simulink model "SM"  (R2023b)
settings: Solver=VariableStepDiscrete  StartTime=0.0  StopTime=2  RelTol=1e-4
values from neighbouring files (symbols this model uses):
  C_PM = 1.758e-3    (= 0.001758)    [HVDCMMCInterconnectionParam.m]
  HRM = 2    [HVDCMMCInterconnectionParam.m]
  L_cable = 15e-3    (= 0.015)    [HVDCMMCInterconnectionParam.m]
  R_cable = 0.5    [HVDCMMCInterconnectionParam.m]
  Tfault = 9999    [HVDCMMCInterconnectionParam.m]
  Ts = Ts_Control    (= 4e-05)    [HVDCMMCInterconnectionParam.m]
  Ts_Power = 20e-6    (= 2e-05)    [HVDCMMCInterconnectionParam.m]
  Vc0_PM = 0    [HVDCMMCInterconnectionParam.m]
  w = 2*pi*Fnom    (= 314.159265359)    [HVDCMMCInterconnectionParam.m]
undefined symbols (not defined in the file or in its folder): DiscIntNeverNeededParam, gcbh, sps_AC, sps_rtmsupport, sps_SM
libraries: simulink x4, spsControlledVoltageSourceLib x3, spsCurrentMeasurementLib x3, spsGroundLib x2, spsDiodeLib x2, spsVoltageMeasurementLib x1, spsThreePhaseSineGeneratorLib x1, spsSeriesRLCBranchLib x1, sps_lib x1
settings Model: Creator=rober  LastModifiedBy=rober

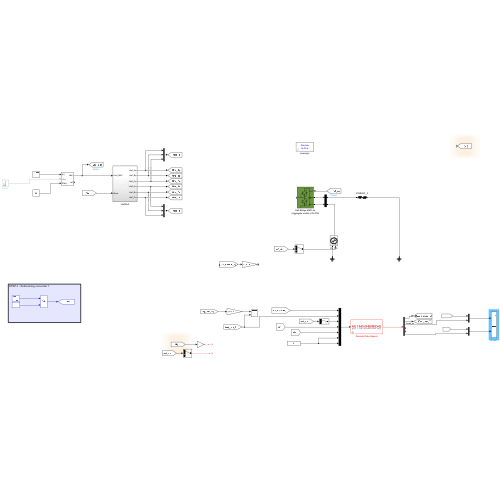
[thumbnail: Simulink's stored preview of the top-level diagram]
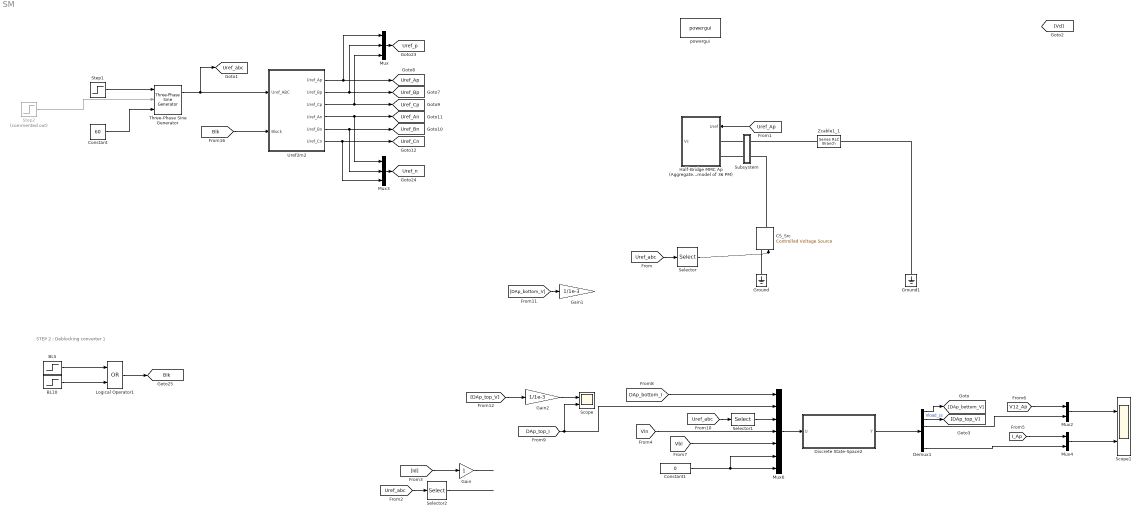
== system SM ==
  note: STEP 2 : Deblocking converter 1
  BL10 : Step  Time=Tfault+Ts_Power  SampleTime=Ts_Power
  BL5 : Step  Time=0.5  Before=1  After=0  SampleTime=Ts_Power
  CS_Src : spsControlledVoltageSourceLib/Controlled Voltage Source  Initialize=on  Source_Type=AC  Amplitude=0  Phase=0  Frequency=0  Measurements=None
  Constant : Constant  Value=60
  Constant1 : Constant  Value=0
  Demux1 : Demux  Outputs=numel(sps_SM.outputs)
  Discrete State-Space2 : Subsystem  SystemSampleTime=Ts_Power  mask{A=sps_SM.A, B=sps_SM.B, C=sps_SM.C, D=sps_SM.D, InitVec=sps_SM.x0, dt=Ts_Power, DQSYM=off, N=HRM, Ws=w}
      mask prompts: InitVec "Initial condition:"; dt "Time step (s):"; N "Harmonic number:"; Ws "Angular frequency (1/rad):"
      mask init:
      | % I = eye(size(A,1));
      | % INVR = I/(I-A*dt/2);
      | % Ad1 = INVR*(I+A*dt/2);
      | % Bd1 = INVR*B*dt/2;
      | % Cd1 = C*Ad1;
      | % Dd11 = C*INVR*B*dt/2+D;
      | % Dd12 = C*INVR*B*dt/2;
      | 
      |     I = eye(size(A,1));
      |     INVR = I/(I-A*dt/2);
      |     Ad1 = INVR*(I+A*dt/2);
      |     Bd1 = INVR*B;
      |     Cd1 = C*INVR*dt;
      |     Dd1 = Cd1*B/2 + D;
      | 
      | DQSYM = get_param(gcb,'DQSYM');
      | 
      | comp = 0;
      | 
      | if(strcmp(DQSYM,'on'))
      | 
      | %Calculating the PNZ matrices
      | 
      |     a = -0.5+0.866i;
      |     a2 = -0.5-0.866i;
      |     Sas = [1,a,a2;1,a2,a;1,1,1]/3;
      | 
      |     arows = size(Ad1,1)/3; %signal size
      |     acols = size(Ad1,2)/3; %signal size
      | 
      |     brows = size(Bd1,1)/3; %signal size
      |     bcols = size(Bd1,2)/3; %signal size
      | 
      |     crows = size(Cd1,1)/3; %signal size
      |     ccols = size(Cd1,2)/3; %signal size
      | 
      |     d1rows = size(Dd1,1)/3; %signal size
      |     d1cols = size(Dd1,2)/3; %signal size
      | 
      |     %%%%%%%%%%%%%%%%%%%%%%% Check for inconsistencies  %%%%%%%%%%%%%%%%%%%%%%%
      | 
      |     szMatA = size(A,1);
      |     iL = eye(szMatA);
      |     szMatiL = size(iL,1);
      | 
      |     if(szMatiL ~= szMatA || size(A,1) ~= size(A,2) || size(iL,1) ~= size(iL,2))
      |         error('[Int_DQN_Mat/swFeedback] check matrix A size!');
      |     end
      | 
      |     if(arows ~= brows || acols ~= ccols || crows ~= d1rows || bcols ~= d1cols)
      |         error('[Int_DQN_Mat/Initialize] the sizes of the state-space matrices!');
      |     end
      | 
      |     %%%%%%%%%%%%%%%%%%%%%%%%%%%%%%%%%%%%%%%%%%%%%%%%%%%%%%%%%%%%%%%
      | 
      | 
      |     %%%%%%%%%%%%%%%%%%%%%%% A --> Bpnz %%%%%%%%%%%%%%%%%%%%%%%
      |     Adc = complex(zeros(3*arows,3*acols));
      | 
      |     for i = 1 : arows
      |         for j = 1 : acols
      |             Adc((1:3) + (i-1)*3,(1:3) + (j-1)*3) = Sas*Ad1((1:3) + (i-1)*3,(1:3) + (j-1)*3)/Sas;
      |             %Adc((1:3) + (i-1)*3,(1:3) + (j-1)*3) = diag(diag(real(Adc((1:3) + (i-1)*3,(1:3) + (j-1)*3))));
      |             %Adc((1:3) + (i-1)*3,(1:3) + (j-1)*3) = diag(diag((Adc((1:3) + (i-1)*3,(1:3) + (j-1)*3))));
      | 
      |         end
      |     end
      |     %%%%%%%%%%%%%%%%%%%%%%%%%%%%%%%%%%%%%%%%%%%%%%%%%%%%%%%%%%%%%%%
      | 
      |     %%%%%%%%%%%%%%%%%%%%%%% B --> Bpnz %%%%%%%%%%%%%%%%%%%%%%%
      | 
      |     Bdc = complex(zeros(3*brows,3*bcols));
      | 
      |     for i = 1 : brows
      |         for j = 1 : bcols
      |             Bdc((1:3) + (i-1)*3,(1:3) + (j-1)*3) = Sas*Bd1((1:3) + (i-1)*3,(1:3) + (j-1)*3)/Sas;
      |             %Bdc((1:3) + (i-1)*3,(1:3) + (j-1)*3) = diag(diag(real(Bdc((1:3) + (i-1)*3,(1:3) + (j-1)*3))));
      |             %Bdc((1:3) + (i-1)*3,(1:3) + (j-1)*3) = diag(diag((Bdc((1:3) + (i-1)*3,(1:3) + (j-1)*3))));
      | 
      |         end
      |     end
      |     %%%%%%%%%%%%%%%%%%%%%%%%%%%%%%%%%%%%%%%%%%%%%%%%%%%%%%%%%%%%%%%
      | 
      |     %%%%%%%%%%%%%%%%%%%%%%% C --> Cpnz %%%%%%%%%%%%%%%%%%%%%%%
      | 
      |     Cdc = complex(zeros(3*crows,3*ccols));
      | 
      |     for i = 1 : crows
      |         for j = 1 : ccols
      |             Cdc((1:3) + (i-1)*3,(1:3) + (j-1)*3) = Sas*Cd1((1:3) + (i-1)*3,(1:3) + (j-1)*3)/Sas;
      |             %Cdc((1:3) + (i-1)*3,(1:3) + (j-1)*3) = diag(diag(real(Cdc((1:3) + (i-1)*3,(1:3) + (j-1)*3))));
      |             %Cdc((1:3) + (i-1)*3,(1:3) + (j-1)*3) = diag(diag((Cdc((1:3) + (i-1)*3,(1:3) + (j-1)*3))));
      |         end
      |     end
      |     %%%%%%%%%%%%%%%%%%%%%%%%%%%%%%%%%%%%%%%%%%%%%%%%%%%%%%%%%%%%%%%
      | 
      |     
      |     %%%%%%%%%%%%%%%%%%%%%%% D1 --> Cpnz %%%%%%%%%%%%%%%%%%%%%%%
      | 
      |     Ddc = complex(zeros(3*d1rows,3*d1cols));
      | 
      |     for i = 1 : d1rows
      |         for j = 1 : d1cols
      |             Ddc((1:3) + (i-1)*3,(1:3) + (j-1)*3) = Sas*Dd1((1:3) + (i-1)*3,(1:3) + (j-1)*3)/Sas;
      |             %Ddc1((1:3) + (i-1)*3,(1:3) + (j-1)*3) = diag(diag(real(Ddc1((1:3) + (i-1)*3,(1:3) + (j-1)*3))));
      |             %Ddc((1:3) + (i-1)*3,(1:3) + (j-1)*3) = diag(diag((Ddc((1:3) + (i-1)*3,(1:3) + (j-1)*3))));
      |         end
      |     end
      |     %%%%%%%%%%%%%%%%%%%%%%%%%%%%%%%%%%%%%%%%%%%%%%%%%%%%%%%%%%%%%%%
      | 
      |     Adc(abs(Adc)<2*eps) = 0;
      |     Bdc(abs(Bdc)<2*eps) = 0;
      |     Cdc(abs(Cdc)<2*eps) = 0;
      |     Ddc(abs(Ddc)<2*eps) = 0;
      | 
      |     InitVec_c = complex(zeros(brows*3,N+1));
      | 
      | 
      |     if(~isempty(InitVec))
      |         if(mod(numel(InitVec),3)~=0) 
      |             warning('[SS_DQNc_Mat] InitVec with wrong size --> needs to be a multiple of 3!'); 
      | 
      |         else
      |             for k = 1 : numel(InitVec)/3
      |                 InitVec_c((k-1)*3+1:(k-1)*3+3,1) = Sas*InitVec((k-1)*3+1:(k-1)*3+3)*exp(+1i*Ws*dt);
      |             end
      |         end
      |     end
      | 
      |     InitVec = InitVec_c;
      | 
      | 
      |     Ad1 = Adc;
      |     Bd1 = Bdc;
      |     Cd1 = Cdc;
      |     Dd1 = Ddc;
      | 
      |     comp = -1i*Ws*dt;
      | 
      | end
      settings: MinAlgLoopOccurrences=on
      settings: LibrarySourceBlock=|
      | spsSynchronousMachineModel/Discrete robust/State Space Model/Discretize
      | BE or Tustin
      mask Callback DQSYM:
      | EMT = get_param(gcb,'DQSYM');
      | 
      | if(strcmp(EMT,'on'))
      |    set_param(gcb,'MaskVisibilities',{'on','on','on','on','on','on','on','on','on'});
      | else
      |    set_param(gcb,'MaskVisibilities',{'on','on','on','on','on','on','on','off','off'});
      | end
      mask Display: disp(['{\color{red}\bf\fontsize{12}x(t) = Ad*x(t-dt)+Bd*u(t)}',newline,'{\color{gray}\bf\fontsize{12}y(t) = Cd*x(t-dt)+Dd*u(t)}'], 'texmode','on');
  Gain : Gain
  Gain1 : Gain  Gain=1/1e-3
  Gain2 : Gain  Gain=1/1e-3
  Ground : spsGroundLib/Ground  LConnTagsString=a
  Ground1 : spsGroundLib/Ground  LConnTagsString=a
  Half-Bridge MMC Ap (Aggregate model of 36 PM) : Subsystem  DialogController=POWERSYS.PowerSysDialog  LoadFcn=sps_rtmsupport('LoadFcn',gcbh);  StartFcn=sps_rtmsupport('StartFcn',gcbh);  StopFcn=sps_rtmsupport('StopFcn',gcbh);  mask(Half-Bridge MMC){ModelType=Aggregate model, n=36, C=C_PM, Vc_Initial=Vc0_PM, Ron=1e-3, Rs=1e6, Cs=inf, Ron_Diode=1e-1, Rs_Diode=1e3, Cs_Diode=inf, Vf_Diode=1e-3, Rs_CurrentSource=inf, Ts=Ts_Power}
      mask prompts: ModelType "Model type:"; n "Number of power modules"; C "Capacitor value (F)"; Vc_Initial "Capacitor initial voltage (V):"; Ron "Device on-state resistance (Ohms)"; Rs "Snubber resistance (Ohms)"; Cs "Snubber capacitance (F)"; Ron_Diode "Diode on-state resistance (Ohms)"; Rs_Diode "Diode snubber resistance (Ohms)"; Cs_Diode "Diode snubber capacitance (F)"; Vf_Diode "Diode forward voltage (V)"; Rs_CurrentSource "Current source snubber resistance (Ohms)"; Ts "Sample time (s):"
      mask help: Implements a half-bridge modular multilevel converter. The converter consists of multiple series-connected power modules. Each power module consists of one half-bridge and one capacitor on the DC side.
      mask init:
      | % block=gcb;
      | % [WantBlockChoice,Index1,MT,SPID] = powericon('FullBridgeMMCInit', block, ModelType, n, Ts, 2);
      | % powericon('SetInternalModels','set',block,WantBlockChoice);
      settings: LibrarySourceBlock=spsHalfBridgeMMCLib/Half-Bridge MMC  CopyFcn=sps_rtmsupport('CopyFcn',gcbh);  DeleteFcn=sps_rtmsupport('DeleteFcn',gcbh);  UndoDeleteFcn=sps_rtmsupport('UndoDeleteFcn',gcbh);  ModelCloseFcn=sps_rtmsupport('ModelCloseFcn',gcbh);  PreSaveFcn=sps_rtmsupport('PreSaveFcn',gcbh);  PostSaveFcn=sps_rtmsupport('PostSaveFcn',gcbh);  NameChangeFcn=sps_rtmsupport('NameChangeFcn',gcbh);  PreCopyFcn=sps_rtmsupport('PreCopyFcn',gcbh);  OpenFcn=sps_rtmsupport('OpenFcn',gcbh, [1]);  CloseFcn=sps_rtmsupport('CloseFcn',gcbh);  PreDeleteFcn=sps_rtmsupport('PreDeleteFcn',gcbh);
      mask Help: helpview(psbhelp);
      mask TypeOptions ModelType: Switching devices | Switching function | Average model (Uref-controlled) | Aggregate model
      mask Callback ModelType: powericon('FullBridgeMMCCback',gcb)
      mask Display:
      | x1=-0.04;
      | plot([0.5 0.80]+x1,[0.95 0.95])
      | plot([0.5 0.5]+x1,[0.95,0.80])
      | plot([0.5 0.38]+x1,[0.80 0.74])
      | plot([0.38 0.38]+x1,[0.80 0.62])
      | plot([0.38 0.5]+x1,[0.68 0.62])
      | plot([0.5 0.5]+x1,[0.62 0.52])
      | plot([0.45 0.5 0.43]+x1,[0.68 0.62 0.60])
      | %
      | y1=0.40;
      | plot([0.5 0.5]+x1,[0.95,0.80]-y1)
      | plot([0.5 0.38]+x1,[0.80 0.74]-y1)
      | plot([0.38 0.38]+x1,[0.80 0.62]-y1)
      | plot([0.38 0.5]+x1,[0.68 0.62]-y1)
      | plot([0.5 0.5]+x1,[0.62 0.52]-y1)
      | plot([0.45 0.5 0.43]+x1,[0.68 0.62 0.60]-y1)
      | plot([0.5 0.5]+x1,[0.2,0.10])
      | plot([0.5 0.80]+x1,[0.1 0.1])
      | %
      | plot([0.5 0.6]+x1,[0.84 0.84])
      | plot([0.6 0.6]+x1,[0.84 0.74])
      | plot([0.6 0.56]+x1,[0.74 0.69])
      | plot([0.6 0.64]+x1,[0.74 0.69])
      | plot([0.56 0.64]+x1,[0.69 0.69])
      | plot([0.6 0.6]+x1,[0.69 0.57])
      | plot([0.5 0.6]+x1,[0.57 0.57])
      | plot([0.55 0.65]+x1,[0.74 0.74])
      | %
      | y2=0.4;
      | plot([0.5 0.6]+x1,[0.84 0.84]-y2)
      | plot([0.6 0.6]+x1,[0.84 0.74]-y2)
      | plot([0.6 0.56]+x1,[0.74 0.69]-y2)
      | plot([0.6 0.64]+x1,[0.74 0.69]-y2)
      | plot([0.56 0.64]+x1,[0.69 0.69]-y2)
      | plot([0.6 0.6]+x1,[0.69 0.57]-y2)
      | plot([0.5 0.6]+x1,[0.57 0.57]-y2)
      | plot([0.55 0.65]+x1,[0.74 0.74]-y2)
      | %
      | plot([0.5 0.23]+x1,[0.5 0.5])
      | plot([0.23 0.23]+x1,[0.5 0.53])
      | plot([0.23 0.23]+x1,[0.55 0.58])
      | plot([0.23 0.23]+x1,[0.61 0.64])
      | %
      | plot([0.5 0.23]+x1,[0.1 0.1])
      | plot([0.23 0.23]+x1,[0.1 0.06])
      | plot([0.23 0.23]+x1,[0.04 0.01])
      | %
      | plot([0.34 0.34]+x1,[0.65 0.75])
      | plot([0.28 0.34]+x1,[0.7 0.7])
      | %
      | plot([0.34 0.34]+x1,[0.65 0.75]-y2)
      | plot([0.28 0.34]+x1,[0.7 0.7]-y2)
      | %
      | % Capacitor
      | plot([0.8 0.8]+x1,[0.51 0.95])
      | plot([0.72 0.88]+x1,[0.51 0.51])
      | plot([0.72 0.88]+x1,[0.51 0.51]-0.04)
      | plot([0.8 0.8]+x1,[0.47 0.1])
      | 
      | color('blue')
      | % switch lower(ModelType)
      | %     case 'average model (uref-controlled)'
      | %         port_label('input',1,'Uref')
      | %     case 'aggregate model'
      | %         port_label('input',1,'Uref')
      | %     otherwise
      | %         port_label('input',1,'Uref')
      | % end
      | port_label('output',1,'m')
  Logical Operator1 : Logic  Operator=OR  AllPortsSameDT=off  OutDataTypeStr=float('double')
  Mux : Mux  Inputs=3
  Mux2 : Mux  Inputs=2
  Mux3 : Mux  Inputs=3
  Mux4 : Mux  Inputs=2
  Mux6 : Mux  Inputs=numel(sps_SM.inputs)
  Scope : Scope  NumInputPorts=2
  Scope1 : Scope  NumInputPorts=2
  Selector : Selector  InputPortWidth=3  IndexOptions=Index vector (dialog)  Indices=1  OutputSizes=1
  Selector1 : Selector  InputPortWidth=3  IndexOptions=Index vector (dialog)  Indices=1  OutputSizes=1
  Selector2 : Selector  InputPortWidth=3  IndexOptions=Index vector (dialog)  Indices=1  OutputSizes=1
  Step1 : Step  Time=0.75  Before=60  After=100  SampleTime=Ts_Power
  Step2 : Step  Commented=on  Time=2.5  After=90  SampleTime=0
  Subsystem : Subsystem
  Three-Phase Sine Generator : spsThreePhaseSineGeneratorLib/Three-Phase Sine Generator  Ts=Ts_Power
      settings: LibrarySourceBlock=|
      | sps_lib/Sources/Signal Generator Sources/Three-Phase
      | Sine Generator
  Uref2m2 : Subsystem
  Zcable1_1 : spsSeriesRLCBranchLib/Series RLC Branch  LConnTagsString=__new0  RConnTagsString=__new0  BranchType=RL  Resistance=R_cable  Inductance=L_cable/3  SetiL0=off  InitialCurrent=0  Capacitance=1e-6  Setx0=off  InitialVoltage=0  Measurements=None
  powergui : sps_lib/powergui  Priority=1  SimulationMode=Discrete  SampleTime=Ts_Power  frequency=60  Iterations=50  frequencyindice=0  Pbase=100e6  ErrMax=1e-4  UnitsV=kV  UnitsW=MW  buscounter=0  FunctionMessages=off  echomessages=off  EnableUseOfTLC=off  CurrentSourceSwitches=off  DisableSnubberDevices=off  DisableRonSwitches=off  DisableVfSwitches=off  DisplayEquations=off  AutomaticDiscreteSolvers=off  SolverType=Tustin/Backward Euler (TBE)  Interpol=off  ExternalGateDelay=off  methode=off  Ts=100  x0status=blocks  SPID=on  SwTol=0  HookPort=off  NonlinearTolerance=1e-4  nMaxIteration=100  ContinueOnMaxIteration=off  RestoreLinks=warning  ResistiveCurrentMeasurement=off  Frange=[0:2:500]  Ylog=off  Xlog=on  ShowGrid=off  save=off  variable=ZData  structure=0  ZoomFFT=off  StartTime=0.0  cycles=1  DisplayStyle=1  fundamental=60  FreqAxis=off  MaxFrequency=1000  frequencyindicesteady=1  RmsSteady=1  display=off
  tag scope: Blk=global, Uref_An=global, Uref_Ap=global, Uref_Bn=global, Uref_Bp=global, Uref_Cn=global, Uref_Cp=global, Uref_abc=global, Uref_n=global, Uref_p=global
  wires:
  [Blk] -> Uref2m2/2(Block)
  Three-Phase Sine Generator/1 -> [Uref_abc], Uref2m2/1(Uref_ABC)
  Step1/1 -> Three-Phase Sine Generator/1
  Constant/1 -> Three-Phase Sine Generator/3
  Logical Operator1/1 -> [Blk]
  BL10/1 -> Logical Operator1/2
  BL5/1 -> Logical Operator1/1
  Uref2m2/6(Uref_Cn) -> Mux3/3, [Uref_Cn]
  Mux3/1 -> [Uref_n]
  Uref2m2/2(Uref_Bp) -> Mux/2, [Uref_Bp]
  Uref2m2/1(Uref_Ap) -> Mux/1, [Uref_Ap]
  Mux/1 -> [Uref_p]
  Uref2m2/5(Uref_Bn) -> Mux3/2, [Uref_Bn]
  Uref2m2/3(Uref_Cp) -> Mux/3, [Uref_Cp]
  Uref2m2/4(Uref_An) -> Mux3/1, [Uref_An]
  [Uref_abc] -> Selector/1
  Selector/1 -> CS_Src/1
  Step2/1 -> Three-Phase Sine Generator/2
  Mux2/1 -> Scope1/1
  Mux4/1 -> Scope1/2
  Mux6/1 -> Discrete State-Space2/1(U)
  Discrete State-Space2/1(Y) -> Demux1/1
  [Uref_Ap] -> Half-Bridge MMC Ap (Aggregate model of 36 PM)/1(Uref)
  Gain/1 -> ?
  [Id] -> Gain/1
  [Uref_abc] -> Selector2/1
  Selector2/1 -> ?
  Constant1/1 -> Mux6/6, Mux6/7
  [DAp_bottom_I] -> Mux6/1
  [DAp_top_I] -> Scope/2, Mux6/2
  [Uref_abc] -> Selector1/1
  [Vin] -> Mux6/4
  [Vbl] -> Mux6/5
  [I_Ap] -> Mux4/1
  Demux1/6 -> Mux4/2
  Demux1/3 -> Mux2/2
  [V12_Ap] -> Mux2/1
  Selector1/1 -> Mux6/3
  Demux1/2 -> [DAp_top_V]  "Vload_ss"
  Demux1/1 -> [DAp_bottom_V]
  [DAp_bottom_V] -> Gain1/1
  [DAp_top_V] -> Gain2/1
  Gain2/1 -> Scope/1
  connections:
  Ground/LConn1 -- CS_Src/LConn1
  Ground1/LConn1 -- Zcable1_1/LConn1
  Zcable1_1/RConn1 -- Subsystem/RConn1
  CS_Src/RConn1 -- Subsystem/RConn2
  Subsystem/LConn1 -- Half-Bridge MMC Ap (Aggregate model of 36 PM)/LConn1
  Subsystem/LConn2 -- Half-Bridge MMC Ap (Aggregate model of 36 PM)/LConn2

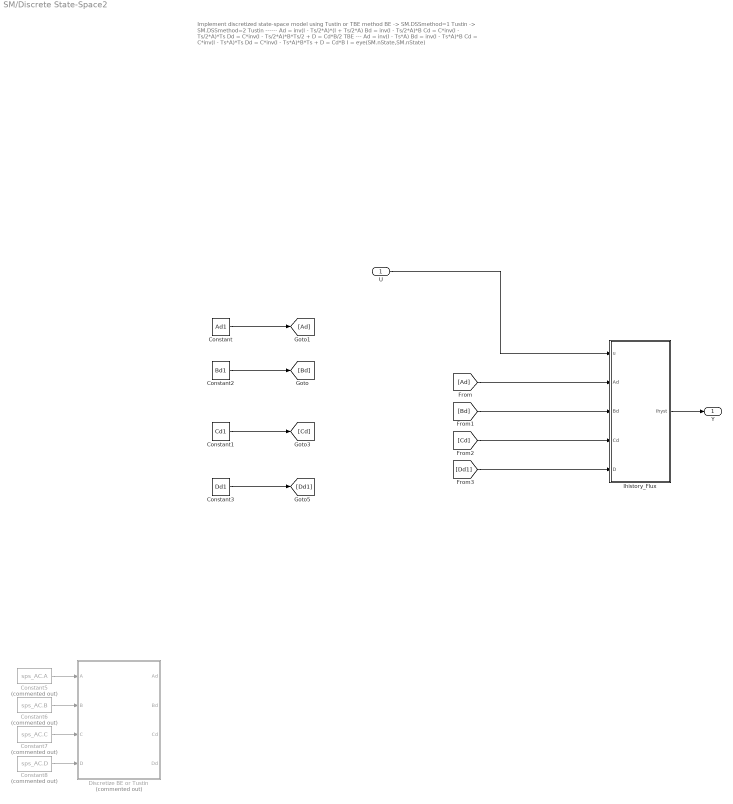
== system SM/Discrete State-Space2 ==
  note: Implement discretized state-space model using Tustin or TBE method
      |
      | BE      -> SM.DSSmethod=1
      | Tustin  -> SM.DSSmethod=2
      |
      |
      | Tustin
      | ------
      | Ad = inv(I - Ts/2*A)*(I + Ts/2*A)
      | Bd = inv(I - Ts/2*A)*B
      | Cd = C*inv(I - Ts/2*A)*Ts
      | Dd = C*inv(I - Ts/2*A)*B*Ts/2  + D  =  Cd*B/2
      |
      | TBE
      | ---
      | Ad = inv(I - Ts*A)
      | Bd = inv(I - Ts*A)*B
      | Cd = C*inv(I - Ts*A)*Ts
      | Dd = C*inv(I - Ts*A)*B*Ts  + D  =  Cd*B
      |
      | I = eye(SM.nState,SM.nState)
  U : Inport
  Constant : Constant  Value=Ad1
  Constant1 : Constant  Value=Cd1
  Constant2 : Constant  Value=Bd1
  Constant3 : Constant  Value=Dd1
  Constant5 : Constant  Commented=on  Value=sps_AC.A
  Constant6 : Constant  Commented=on  Value=sps_AC.B
  Constant7 : Constant  Commented=on  Value=sps_AC.C
  Constant8 : Constant  Commented=on  Value=sps_AC.D
  Discretize BE or Tustin : Subsystem  Commented=on  AncestorBlock="DQN_Machines/DQN_Mac_V1/Discretize  BE or Tustin"
  Ihistory_Flux : Subsystem  AncestorBlock=DQN_Machines/DQN_Mac_V1/Ihistory_Flux
  Y : Outport
  wires:
  Constant/1 -> [Ad]
  Constant2/1 -> [Bd]
  Constant1/1 -> [Cd]
  Constant3/1 -> [Dd1]
  Constant7/1 -> Discretize BE or Tustin/3(C)
  Constant6/1 -> Discretize BE or Tustin/2(B)
  Constant8/1 -> Discretize BE or Tustin/4(D)
  Constant5/1 -> Discretize BE or Tustin/1(A)
  U/1 -> Ihistory_Flux/1(u)
  Ihistory_Flux/1(Ihyst) -> Y/1
  [Ad] -> Ihistory_Flux/2(Ad)
  [Bd] -> Ihistory_Flux/3(Bd)
  [Cd] -> Ihistory_Flux/4(Cd)
  [Dd1] -> Ihistory_Flux/5(D)

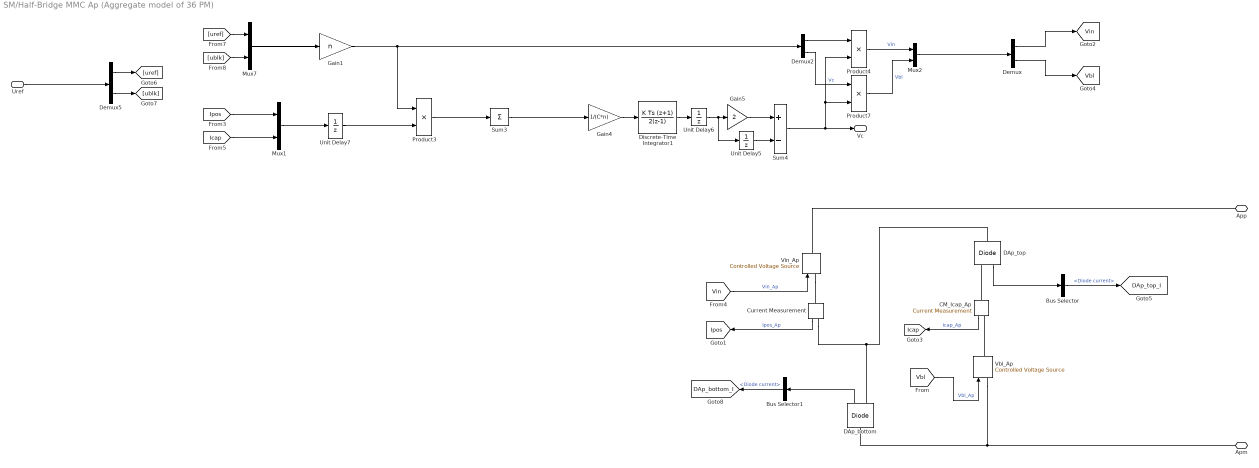
== system SM/Half-Bridge MMC Ap (Aggregate model of 36 PM) ==
  Uref : Inport
  Bus Selector : BusSelector  OutputSignals=Diode current
  Bus Selector1 : BusSelector  OutputSignals=Diode current
  CM_Icap_Ap : spsCurrentMeasurementLib/Current Measurement  PhasorSimulation=off  OutputType=Complex  PSBequivalent=0
  Current Measurement : spsCurrentMeasurementLib/Current Measurement  PhasorSimulation=off  OutputType=Complex  PSBequivalent=0
  DAp_bottom : spsDiodeLib/Diode  Ron=0.0001  Lon=0  Vf=0.0001  IC=0  UseSnubber=0  Rs=1e9  Cs=Cs_Diode  Measurements=on
  DAp_top : spsDiodeLib/Diode  Ron=0.0001  Lon=0  Vf=0.0001  IC=0  UseSnubber=0  Rs=1e9  Cs=Cs_Diode  Measurements=on
  Demux : Demux  Outputs=2
  Demux2 : Demux  Outputs=2
  Demux5 : Demux  Outputs=2
  Discrete-Time Integrator1 : DiscreteIntegrator  IntegratorMethod=Integration: Trapezoidal  gainval=1  InitialCondition=Vc_Initial  SampleTime=Ts  UpperSaturationLimit=5000  LowerSaturationLimit=500  ICPrevOutput=DiscIntNeverNeededParam  ICPrevScaledInput=DiscIntNeverNeededParam
  Gain1 : Gain  Gain=n
  Gain4 : Gain  Gain=1/(C*n)
  Gain5 : Gain  Gain=2
  Mux1 : Mux  Inputs=2
  Mux2 : Mux  Inputs=2
  Mux7 : Mux  Inputs=2
  Product3 : Product
  Product4 : Product
  Product7 : Product
  Sum3 : Sum  Inputs=1  InputSameDT=on  SaturateOnIntegerOverflow=on  OutDataTypeStr=Inherit: Same as first input
  Sum4 : Sum  Inputs=+-  InputSameDT=on  SaturateOnIntegerOverflow=on  OutDataTypeStr=Inherit: Same as first input
  Unit Delay5 : UnitDelay  InitialCondition=Vc_Initial  SampleTime=Ts  HasFrameUpgradeWarning=on
  Unit Delay6 : UnitDelay  InitialCondition=Vc_Initial  SampleTime=Ts  HasFrameUpgradeWarning=on
  Unit Delay7 : UnitDelay  SampleTime=Ts  HasFrameUpgradeWarning=on
  Vbl_Ap : spsControlledVoltageSourceLib/Controlled Voltage Source  Initialize=on  Source_Type=AC  Amplitude=0  Phase=0  Frequency=0  Measurements=None
  Vin_Ap : spsControlledVoltageSourceLib/Controlled Voltage Source  Initialize=on  Source_Type=AC  Amplitude=0  Phase=0  Frequency=0  Measurements=None
  App : PMIOPort  Side=Left
  Apm : PMIOPort  Port=2  Side=Left
  Vc : Outport  VectorParamsAs1DForOutWhenUnconnected=off
  tag scope: DAp_bottom_I=global, DAp_top_I=global, Icap=global, Ipos=global, Vbl=global, Vin=global
  wires:
  Demux/1 -> [Vin]
  [Vin] -> Vin_Ap/1  "Vin_Ap"
  Product3/1 -> Sum3/1
  Demux/2 -> [Vbl]
  [Ipos] -> Mux1/1
  Unit Delay5/1 -> Sum4/2
  Gain5/1 -> Sum4/1
  Sum4/1 -> Product7/2, Product4/2, Vc/1  "Vc"
  Discrete-Time Integrator1/1 -> Unit Delay6/1
  Mux2/1 -> Demux/1
  [Vbl] -> Vbl_Ap/1  "Vbl_Ap"
  [Icap] -> Mux1/2
  Gain4/1 -> Discrete-Time Integrator1/1
  Unit Delay6/1 -> Gain5/1, Unit Delay5/1
  Mux1/1 -> Unit Delay7/1
  Mux7/1 -> Gain1/1
  Demux2/1 -> Product4/1
  Demux2/2 -> Product7/1
  Product4/1 -> Mux2/1  "Vin"
  Product7/1 -> Mux2/2  "Vbl"
  Demux5/2 -> [ublk]
  [uref] -> Mux7/1
  [ublk] -> Mux7/2
  Current Measurement/1 -> [Ipos]  "Ipos_Ap"
  CM_Icap_Ap/1 -> [Icap]  "Icap_Ap"
  Unit Delay7/1 -> Product3/2
  Gain1/1 -> Demux2/1, Product3/1
  Demux5/1 -> [uref]
  Uref/1 -> Demux5/1
  Sum3/1 -> Gain4/1
  DAp_top/1 -> Bus Selector/1
  Bus Selector/1 -> [DAp_top_I]  "<Diode current>"
  DAp_bottom/1 -> Bus Selector1/1
  Bus Selector1/1 -> [DAp_bottom_I]  "<Diode current>"
  connections:
  Current Measurement/RConn1 -- DAp_bottom/RConn1 -- DAp_top/LConn1
  Apm/RConn1 -- Vbl_Ap/LConn1 -- DAp_bottom/LConn1
  Vbl_Ap/RConn1 -- CM_Icap_Ap/RConn1
  CM_Icap_Ap/LConn1 -- DAp_top/RConn1
  App/RConn1 -- Vin_Ap/RConn1
  Vin_Ap/LConn1 -- Current Measurement/LConn1

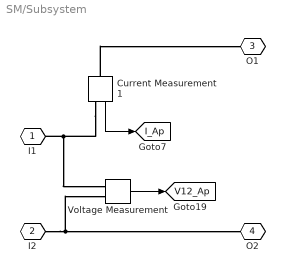
== system SM/Subsystem ==
  Current Measurement1 : spsCurrentMeasurementLib/Current Measurement  PhasorSimulation=off  OutputType=Complex  PSBequivalent=0
  Voltage Measurement : spsVoltageMeasurementLib/Voltage Measurement  PhasorSimulation=off  OutputType=Complex  PSBequivalent=0
  I1 : PMIOPort  Side=Left
  I2 : PMIOPort  Port=2  Side=Left
  O1 : PMIOPort  Port=3  Side=Right
  O2 : PMIOPort  Port=4  Side=Right
  tag scope: I_Ap=global, V12_Ap=global
  wires:
  Current Measurement1/1 -> [I_Ap]
  Voltage Measurement/1 -> [V12_Ap]
  connections:
  Current Measurement1/RConn1 -- Voltage Measurement/LConn1 -- I1/RConn1
  Current Measurement1/LConn1 -- O1/RConn1
  I2/RConn1 -- Voltage Measurement/LConn2 -- O2/RConn1

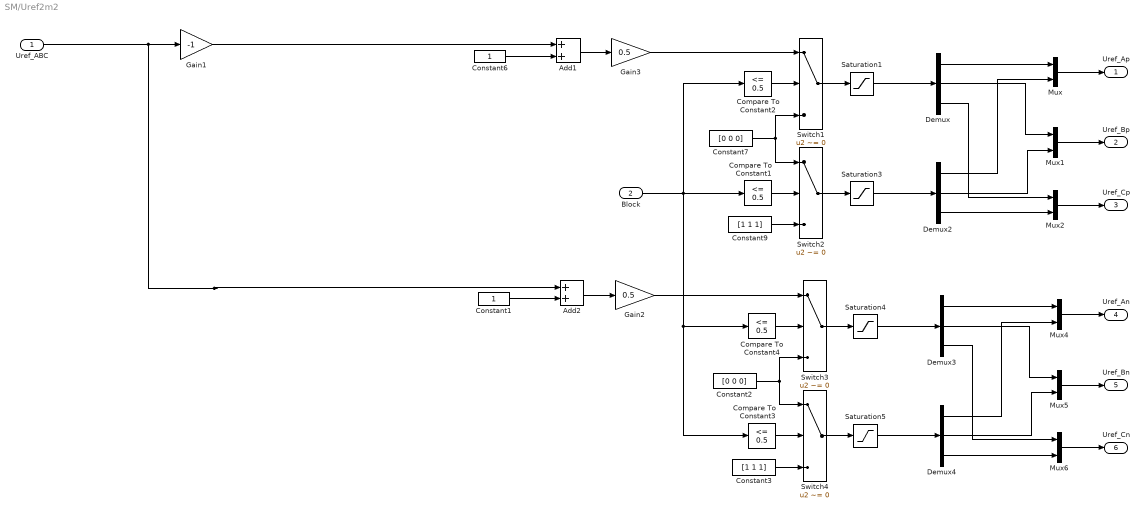
== system SM/Uref2m2 ==
  Uref_ABC : Inport  PortDimensions=3
  Block : Inport  Port=2
  Add1 : Sum
  Add2 : Sum
  Compare To Constant{1..4} (4 alike) : simulink/Logic and Bit Operations/Compare To Constant  relop=<=  const=0.5  OutDataTypeStr=boolean
  Constant1 : Constant
  Constant2 : Constant  Value=[0 0 0]
  Constant3 : Constant  Value=[1 1 1]
  Constant6 : Constant
  Constant7 : Constant  Value=[0 0 0]
  Constant9 : Constant  Value=[1 1 1]
  Demux{,2..4} (4 alike) : Demux  Outputs=3
  Gain1 : Gain  Gain=-1
  Gain2 : Gain  Gain=0.5
  Gain3 : Gain  Gain=0.5
  Mux{,1..2,4..6} (6 alike) : Mux  Inputs=2
  Saturation{1,3..5} (4 alike) : Saturate  UpperLimit=1  LowerLimit=0
  Switch{1..4} (4 alike) : Switch  Criteria=u2 ~= 0  SaturateOnIntegerOverflow=off  InputSameDT=off
  Uref_Ap : Outport
  Uref_Bp : Outport  Port=2
  Uref_Cp : Outport  Port=3
  Uref_An : Outport  Port=4
  Uref_Bn : Outport  Port=5
  Uref_Cn : Outport  Port=6
  wires:
  Add1/1 -> Gain3/1
  Gain3/1 -> Switch1/1
  Constant7/1 -> Switch1/3, Switch2/1
  Compare To Constant1/1 -> Switch2/2
  Constant6/1 -> Add1/2
  Constant9/1 -> Switch2/3
  Compare To Constant2/1 -> Switch1/2
  Gain1/1 -> Add1/1
  Mux/1 -> Uref_Ap/1
  Switch1/1 -> Saturation1/1
  Switch2/1 -> Saturation3/1
  Demux/1 -> Mux/1
  Demux2/1 -> Mux/2
  Demux/2 -> Mux1/1
  Demux2/2 -> Mux1/2
  Demux2/3 -> Mux2/2
  Demux/3 -> Mux2/1
  Demux4/1 -> Mux4/2
  Demux4/2 -> Mux5/2
  Constant1/1 -> Add2/2
  Compare To Constant4/1 -> Switch3/2
  Compare To Constant3/1 -> Switch4/2
  Add2/1 -> Gain2/1
  Constant2/1 -> Switch3/3, Switch4/1
  Block/1 -> Compare To Constant1/1, Compare To Constant4/1, Compare To Constant3/1, Compare To Constant2/1
  Uref_ABC/1 -> Add2/1, Gain1/1
  Switch3/1 -> Saturation4/1
  Demux3/2 -> Mux5/1
  Demux3/3 -> Mux6/1
  Constant3/1 -> Switch4/3
  Demux3/1 -> Mux4/1
  Switch4/1 -> Saturation5/1
  Gain2/1 -> Switch3/1
  Demux4/3 -> Mux6/2
  Saturation1/1 -> Demux/1
  Saturation3/1 -> Demux2/1
  Saturation4/1 -> Demux3/1
  Saturation5/1 -> Demux4/1
  Mux1/1 -> Uref_Bp/1
  Mux2/1 -> Uref_Cp/1
  Mux4/1 -> Uref_An/1
  Mux5/1 -> Uref_Bn/1
  Mux6/1 -> Uref_Cn/1

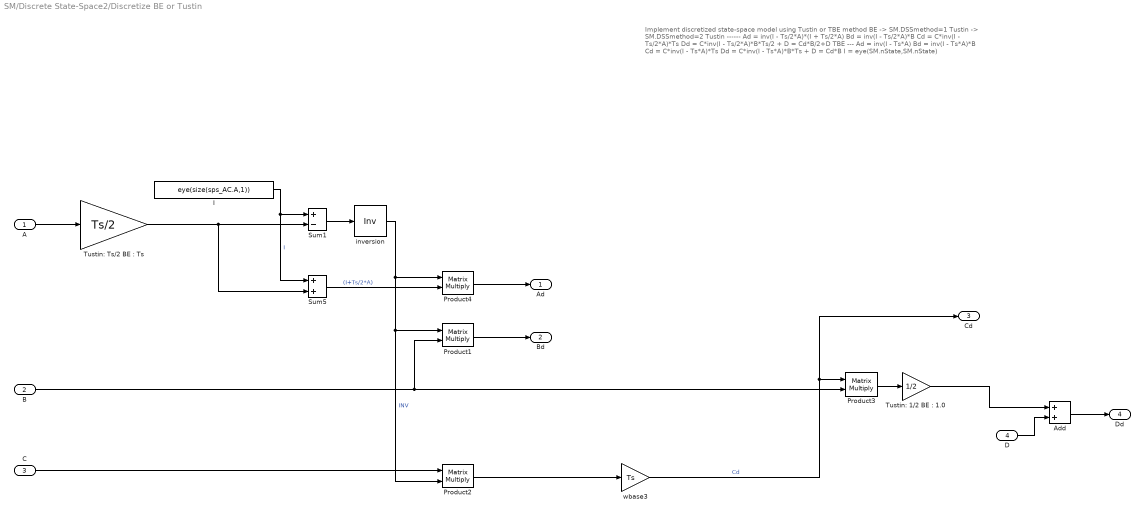
== system SM/Discrete State-Space2/Discretize BE or Tustin ==
  note: Implement discretized state-space model using Tustin or TBE method
      |
      | BE      -> SM.DSSmethod=1
      | Tustin  -> SM.DSSmethod=2
      |
      |
      | Tustin
      | ------
      | Ad = inv(I - Ts/2*A)*(I + Ts/2*A)
      | Bd = inv(I - Ts/2*A)*B
      | Cd = C*inv(I - Ts/2*A)*Ts
      | Dd = C*inv(I - Ts/2*A)*B*Ts/2  + D  =  Cd*B/2+D
      |
      | TBE
      | ---
      | Ad = inv(I - Ts*A)
      | Bd = inv(I - Ts*A)*B
      | Cd = C*inv(I - Ts*A)*Ts
      | Dd = C*inv(I - Ts*A)*B*Ts  + D  =  Cd*B
      |
      | I = eye(SM.nState,SM.nState)
  A : Inport
  B : Inport  Port=2
  C : Inport  Port=3
  D : Inport  Port=4
  Add : Sum
  I : Constant  Value=eye(size(sps_AC.A,1))
  Product{1..4} (4 alike) : Product  Multiplication=Matrix(*)  SaturateOnIntegerOverflow=on  OutDataTypeStr=Inherit: Same as first input
  Sum1 : Sum  Inputs=+-  SaturateOnIntegerOverflow=on
  Sum5 : Sum  SaturateOnIntegerOverflow=on
  "Tustin: 1/2 BE : 1.0" : Gain  Gain=1/2  SaturateOnIntegerOverflow=on  OutDataTypeStr=Inherit: Same as input  ParamDataTypeStr=Inherit: Same as input
  "Tustin: Ts/2 BE : Ts" : Gain  Gain=Ts/2  SaturateOnIntegerOverflow=on  OutDataTypeStr=Inherit: Same as input  ParamDataTypeStr=Inherit: Same as input
  inversion : Product  Inputs=/  Multiplication=Matrix(*)  RndMeth=Zero
  wbase3 : Gain  Gain=Ts  SaturateOnIntegerOverflow=on  OutDataTypeStr=Inherit: Same as input  ParamDataTypeStr=Inherit: Same as input
  Ad : Outport  VectorParamsAs1DForOutWhenUnconnected=off
  Bd : Outport  Port=2  VectorParamsAs1DForOutWhenUnconnected=off
  Cd : Outport  Port=3  VectorParamsAs1DForOutWhenUnconnected=off
  Dd : Outport  Port=4  VectorParamsAs1DForOutWhenUnconnected=off
  wires:
  wbase3/1 -> Product3/1, Cd/1  "Cd"
  Product2/1 -> wbase3/1
  "Tustin: 1/2 BE : 1.0"/1 -> Add/1
  Product3/1 -> "Tustin: 1/2 BE : 1.0"/1
  C/1 -> Product2/1
  B/1 -> Product3/2, Product1/2
  Product1/1 -> Bd/1
  Sum5/1 -> Product4/2  "(I+Ts/2*A)"
  inversion/1 -> Product4/1, Product1/1, Product2/2  "INV"
  Sum1/1 -> inversion/1
  I/1 -> Sum1/1, Sum5/1  "I"
  A/1 -> "Tustin: Ts/2 BE : Ts"/1
  Product4/1 -> Ad/1
  "Tustin: Ts/2 BE : Ts"/1 -> Sum5/2, Sum1/2
  Add/1 -> Dd/1
  D/1 -> Add/2

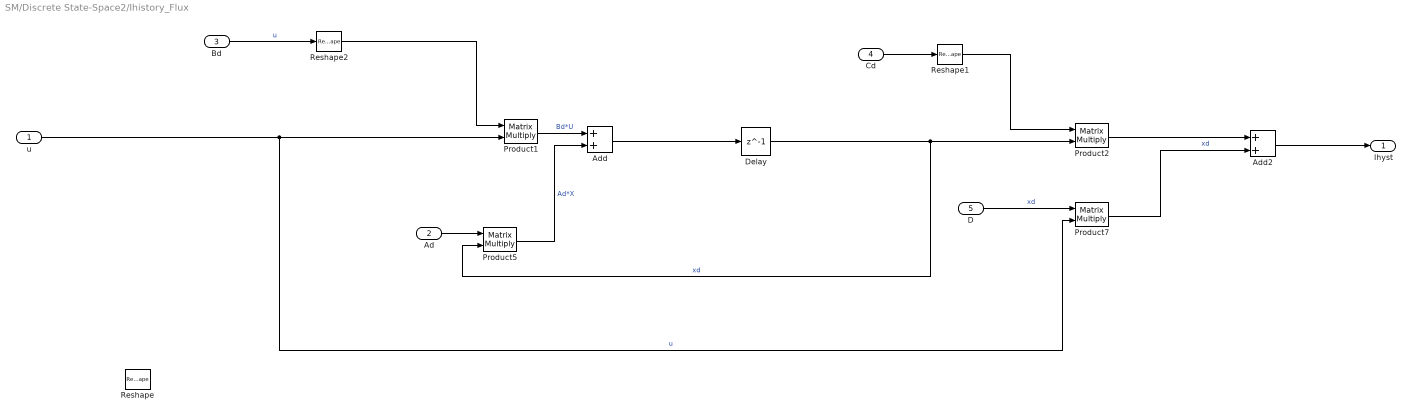
== system SM/Discrete State-Space2/Ihistory_Flux ==
  u : Inport
  Ad : Inport  Port=2
  Bd : Inport  Port=3
  Cd : Inport  Port=4
  D : Inport  Port=5
  Add : Sum
  Add2 : Sum
  Delay : Delay  DelayLength=1  InitialCondition=InitVec  SampleTime=dt
  Product{1..2,5,7} (4 alike) : Product  Multiplication=Matrix(*)  SaturateOnIntegerOverflow=on  OutDataTypeStr=Inherit: Same as first input
  Reshape : Reshape
  Reshape1 : Reshape  OutputDimensionality=Customize  OutputDimensions=[6,1]
  Reshape2 : Reshape  OutputDimensionality=Customize  OutputDimensions=[1,7]
  Ihyst : Outport  VectorParamsAs1DForOutWhenUnconnected=off
  wires:
  Add2/1 -> Ihyst/1
  Bd/1 -> Reshape2/1  "u"
  u/1 -> Product7/2, Product1/2  "u"
  Product2/1 -> Add2/1
  Product1/1 -> Add/1  "Bd*U"
  Add/1 -> Delay/1
  Delay/1 -> Product2/2, Product5/2  "xd"
  Product5/1 -> Add/2  "Ad*X"
  Ad/1 -> Product5/1
  Product7/1 -> Add2/2  "xd"
  D/1 -> Product7/1  "xd"
  Cd/1 -> Reshape1/1
  Reshape1/1 -> Product2/1
  Reshape2/1 -> Product1/1
